simulink model "LinearSim"  (R2018b)
settings: Solver=ode45  StartTime=0.0  StopTime=15  RelTol=1e-3  EnableMultiTasking=on
values from neighbouring files (symbols this model uses):
  A = [0.2    1.2  -10 ... (first row only)    [example.m]    (also in linearized_control.m = [zeros(2,2) eye(2);-Mbar\Kbar -Mbar\Fbar]; observer.m = [zeros(2,2) eye(2);-Mbar\Kbar -Mbar\Fbar]; observerSFunction.m = [zeros(2,2) eye(2);-Mbar\Kbar -Mbar\Fbar]; sfunc.m)
  B = [1,-1 ... (first row only)    [example.m]    (also in linearized_control.m = [zeros(2,2);inv(Mbar)]*[1;0]; observer.m = [zeros(2,2);inv(Mbar)]*[1;0]; observerSFunction.m = [zeros(2,2);inv(Mbar)]*[1;0]; sfunc.m)
  K = place(A,B,Pd)    [linearized_control.m]
  X0 = [q10-0.1, q20+.2 , 0 ,0]'    [linearized_control.m]
settings Model: Creator=amiria  LastModifiedBy=AndyA
settings DataIOCC: LimitDataPoints=on  SaveFormat=Array
settings OptimizationCC: ExpressionDepthLimit=2147483647  LifeSpan=inf
settings DebuggingCC: UnderspecifiedInitializationDetection=Classic  MergeDetectMultiDrivingBlocksExec=none  SolverPrmCheckMsg=warning  StateNameClashWarn=warning  SFUnexpectedBacktrackingDiag=warning  SFNoUnconditionalDefaultTransitionDiag=warning  SFExecutionAtInitializationDiag=none
settings HardwareCC: ProdBitPerPointer=32  ProdBitPerSizeT=32  ProdBitPerPtrDiffT=32  ProdLargestAtomicFloat=None  ProdIntDivRoundTo=Undefined  ProdEndianess=Unspecified  ProdWordSize=32  ProdHWDeviceType=32-bit Generic
settings ModelReferenceCC: PropagateSignalLabelsOutOfModel=off
settings SFSimCC: SimUseLocalCustomCode=off
settings RTWCC: RTWUseLocalCustomCode=off
settings CodeAppCC: StateflowObjectComments=on
settings GRTTargetCC: TargetLangStandard=C89/C90 (ANSI)  GeneratePreprocessorConditionals=Disable all
settings ConfigComp: CovMetricSettings=dw  CovHtmlReporting=on  CovSaveCumulativeToWorkspaceVar=on  CovSaveSingleToWorkspaceVar=on  CovExternalEMLEnable=off

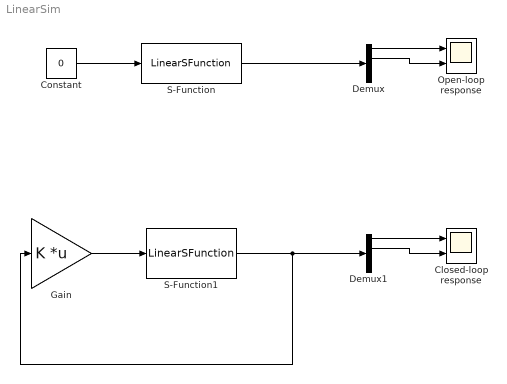
== system LinearSim ==
  Closed-loop response : Scope  NumInputPorts=2
  Constant : Constant  Value=0
  Demux : Demux
  Demux1 : Demux
  Gain : Gain  Gain=K  Multiplication=Matrix(K*u)
  "Open-loop response " : Scope  NumInputPorts=2
  S-Function : S-Function  FunctionName=LinearSFunction  Parameters=X0,A,B  SFunctionDeploymentMode=off  EnableBusSupport=off
  S-Function1 : S-Function  FunctionName=LinearSFunction  Parameters=X0,A,B  SFunctionDeploymentMode=off  EnableBusSupport=off
  wires:
  Demux/1 -> "Open-loop response "/1
  Demux/2 -> "Open-loop response "/2
  S-Function/1 -> Demux/1
  Gain/1 -> S-Function1/1
  Demux1/1 -> Closed-loop response/1
  Demux1/2 -> Closed-loop response/2
  S-Function1/1 -> Gain/1, Demux1/1
  Constant/1 -> S-Function/1
